simulink model "controlNoLinealBloques"  (R2023b)
settings: Solver=VariableStepAuto  StartTime=0.0  StopTime=10.0  RelTol=1e-3
values from neighbouring files (symbols this model uses):
  qc = robot.ikine(Tcart,q0,'mask',mask)    [TP_2.m]
libraries: roblocks x7
settings Model: Creator=nmestanza  LastModifiedBy=nmestanza

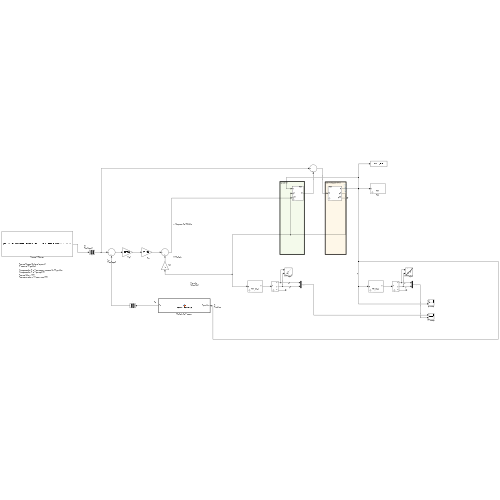
[thumbnail: Simulink's stored preview of the top-level diagram]
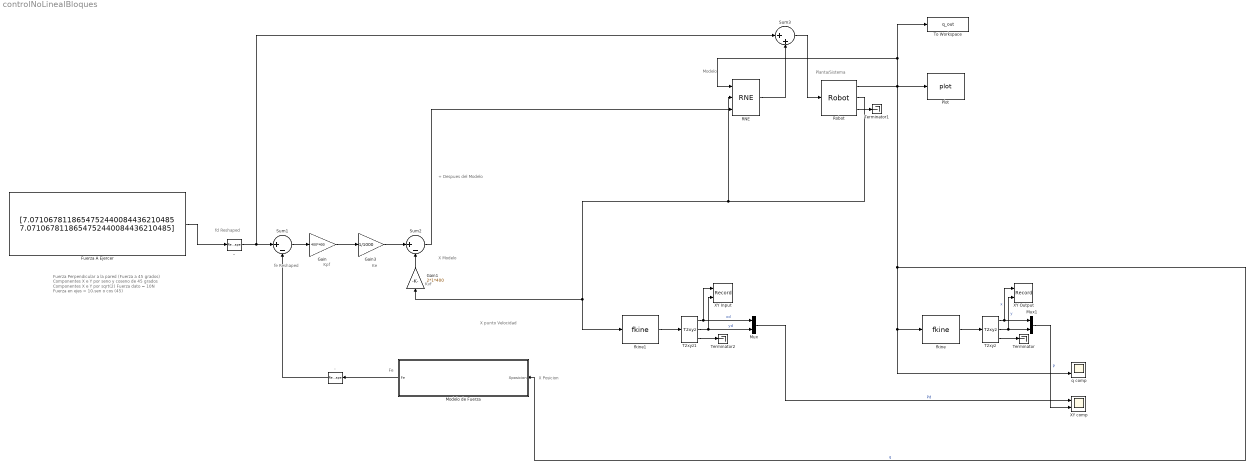
== system controlNoLinealBloques ==
  note: Modelo
  note: Planta/Sistema
  note: Fe
  note: Kpf
  note: Kvf
  note: Fuerza Perpendicular a la pared
      | (Fuerza a 45 grados)
      |
      | Componentes X e Y por seno y coseno de 45 grados
      | Componentes X e Y por sqrt(2)
      |
      | Fuerza dato = 10N
      | Fuerza en ejes = 10.sen o cos (45)
  note: fd
      | Reshaped
  note: X Modelo
  note: X
      | Posicion
  note: Ke
  note: X punto
      | Velocidad
  note: fe
      | Reshaped
  note: + Despues del Modelo
  . : Reshape  OutputDimensionality=Column vector (2-D)
  .. : Reshape  OutputDimensionality=Column vector (2-D)
  Fuerza A Ejercer : Constant  Value=[7.0710678118654752440084436210485 7.0710678118654752440084436210485]
  Gain : Gain  Gain=400*400
  Gain1 : Gain  Gain=2*1*400
  Gain3 : Gain  Gain=1/1000
  Modelo de Fuerza : MATLAB Function  TreatAsAtomicUnit=on
  Mux : Mux  Inputs=2
  Mux1 : Mux  Inputs=2
  Plot : roblocks/Arm/plot  robot=robot  fps=25  holdplot=on
  RNE : roblocks/Arm/RNE  robot=robot  grav=[0 0 9.81]
  Robot : roblocks/Arm/Robot  robot=robot  q0=qc(1,:)
  Sum1 : Sum  Inputs=|+-
  Sum2 : Sum  Inputs=|+-
  Sum3 : Sum  Inputs=|++
  T2xyz : roblocks/Toolbox/T2xyz
  T2xyz1 : roblocks/Toolbox/T2xyz
  Terminator : Terminator
  Terminator1 : Terminator
  Terminator2 : Terminator
  To Workspace : ToWorkspace  VariableName=q_out  SaveFormat=Timeseries  SampleTime=-1
  XY Input : Record  FileSettingsInternal="{\"entries\":[{\"content\":{\"excelSettings\":{\"content\":{},\"type\":\"Streamout.ExcelSettings\"}},\"type\":\"Streamout.FileSettingStorage\",\"uuid\":\"\"}],\"packageUris\":[\"http:\\/\\/schema.mathworks.com\\/mf0\\/streamout_blocks\\/R2020a\"],\"version\":\"1.0\"}"  Layout=[1 1]  SignalsInternal="{\"entries\":[{\"content\":{\"signals\":[{\"content\":{\"blockPath\":[],\"dimensions\":[1],\"domain\":\"\",\"lineColor\":\"#a2142f\",\"plots\":[1],\"port\":1,\"sid\":[\"\"],\"signalID\":133,\"signalName\":\"xd\"},\"type\":\"RecordBlkView.Signal\",\"uuid\":\"\"},{\"content\":{\"blockPath\":[],\"dimensions\":[1],\"domain\":\"\",\"lineColor\":\"#139fff\",\"plots\":[1],\"port\":2,\"sid\":[\"\"],\"signalID\":137,\"signalName\":\"yd\"},\"type\":\"RecordBlkView.Signal\",\"uuid\":\"\"}]},\"type\":\"RecordBlkView.InputSignals\",\"uuid\":\"\"}],\"packageUris\":[\"http:\\/\\/schema.mathworks.com\\/mf0\\/streamout_blocks\\/R2020a\"],\"version\":\"1.0\"}"  VisualizationBindings="{\"xyplotplugin\":{\"info\":[{\"series\":[{\"bindingParametersList\":[{\"parameter\":\"X-Axis\",\"signalID\":133,\"signalName\":\"xd\"},{\"parameter\":\"Y-Axis\",\"signalID\":137,\"signalName\":\"yd\"}],\"seriesID\":50006}],\"subplotID\":1}]}}"  CompatibilityTag=XY  st=-1
  XY Output : Record  FileSettingsInternal="{\"entries\":[{\"content\":{\"excelSettings\":{\"content\":{},\"type\":\"Streamout.ExcelSettings\"}},\"type\":\"Streamout.FileSettingStorage\",\"uuid\":\"\"}],\"packageUris\":[\"http:\\/\\/schema.mathworks.com\\/mf0\\/streamout_blocks\\/R2020a\"],\"version\":\"1.0\"}"  Layout=[1 1]  SignalsInternal="{\"entries\":[{\"content\":{\"signals\":[{\"content\":{\"blockPath\":[],\"dimensions\":[1],\"domain\":\"\",\"lineColor\":\"#a2142f\",\"plots\":[1],\"port\":1,\"sid\":[\"\"],\"signalID\":141,\"signalName\":\"x\"},\"type\":\"RecordBlkView.Signal\",\"uuid\":\"\"},{\"content\":{\"blockPath\":[],\"dimensions\":[1],\"domain\":\"\",\"lineColor\":\"#139fff\",\"plots\":[1],\"port\":2,\"sid\":[\"\"],\"signalID\":145,\"signalName\":\"y\"},\"type\":\"RecordBlkView.Signal\",\"uuid\":\"\"}]},\"type\":\"RecordBlkView.InputSignals\",\"uuid\":\"\"}],\"packageUris\":[\"http:\\/\\/schema.mathworks.com\\/mf0\\/streamout_blocks\\/R2020a\"],\"version\":\"1.0\"}"  VisualizationBindings="{\"xyplotplugin\":{\"info\":[{\"series\":[{\"bindingParametersList\":[{\"parameter\":\"X-Axis\",\"signalID\":141,\"signalName\":\"x\"},{\"parameter\":\"Y-Axis\",\"signalID\":145,\"signalName\":\"y\"}],\"seriesID\":38420}],\"subplotID\":1}]}}"  CompatibilityTag=XY  st=-1
  XY comp : Scope  NumInputPorts=2
  fkine : roblocks/Arm/fkine  robot=robot_dis
  fkine1 : roblocks/Arm/fkine  robot=robot_dis
  q comp : Scope  NumInputPorts=2
  wires:
  fkine/1 -> T2xyz/1
  T2xyz/3 -> Terminator/1
  T2xyz/2 -> Mux1/2, XY Output/2  "y"
  Robot/1 -> RNE/1, To Workspace/1, Modelo de Fuerza/1(Xposicion), fkine/1, q comp/2, Plot/1  "q"
  Robot/2 -> fkine1/1, Gain1/1, RNE/2
  T2xyz1/3 -> Terminator2/1
  T2xyz/1 -> XY Output/1, Mux1/1  "x"
  T2xyz1/1 -> XY Input/1, Mux/1  "xd"
  T2xyz1/2 -> XY Input/2, Mux/2  "yd"
  fkine1/1 -> T2xyz1/1
  Robot/3 -> Terminator1/1
  Mux1/1 -> XY comp/2  "P"
  Mux/1 -> XY comp/1  "Pd"
  ./1 -> Sum1/2
  Modelo de Fuerza/1(Fe) -> ./1
  ../1 -> Sum3/1, Sum1/1
  Sum1/1 -> Gain/1
  Fuerza A Ejercer/1 -> ../1
  Gain3/1 -> Sum2/1
  Gain1/1 -> Sum2/2
  Gain/1 -> Gain3/1
  Sum2/1 -> RNE/3
  RNE/1 -> Sum3/2
  Sum3/1 -> Robot/1

== matlab function controlNoLinealBloques/Modelo de Fuerza ==
  data: Xposicion input; Fe output
%Input: Vector de coordenadas bidimensionales Xposicion como entrada
%Output: Vector de fuerzas bidimensionales Fe 

%Description: Evalar la posición del punto representado por las coordenadas 
%Xposicion con respecto a la pared 
%En base a ello, calcula la fuerza correspondiente.

function Fe = modeloFuerzaCalc(Xposicion)

kEnv = 1000; %N/mm
ejeY = Xposicion(2);
ejeX = Xposicion(1);

%Pared interseca el plano XY en una línea que contiene los puntos (2; 0) y (0; 2)
%Verification Total:
%limY = (ejeX*(-1)+2)/1 = 2 - ejeX
%limX = ((ejeY*1)-2)/-1 = 2 - ejeY
%Por ende:
%ejeX < limX y ejeY< limY
%ejeY < 2 - ejeX ; ejeX < 2 - ejeY
%ejeY + ejeX - 2 + ejeX + ejeY  -2 < 0 
%2ejeX + 2ejeY - 4 < 0 -> ejeX + ejeY - 2 < 0

%Verifico si el punto está en el lado negativo de la pared
%Calculo la distancia entre el punto y la pared
%Defino la fuerza en función de esa distancia.

if (2-ejeX-ejeY) <= 0 

    distancia = abs(2-ejeX-ejeY)/sqrt(1^2+1^2);
    Fe = [distancia*kEnv*sqrt(2)/2, distancia*kEnv*sqrt(2)/2];

%Verifico si el punto está en el lado positivo de la pared 

else 

    Fe=[0, 0];



end
